simulink model "TLfaultDetection"  (R2024b)
settings: Solver=VariableStepAuto  StartTime=0.0  StopTime=0.15  RelTol=1e-3
undefined symbols (not defined in the file or in its folder): D1, Delta
libraries: spsCurrentMeasurementLib x4, spsDistributedParametersLineLib x2, spsThreePhaseVIMeasurementLib x2, spsThreePhaseParallelRLCLoadLib x1, spsThreePhaseTransformerTwoWindingsLib x1, spsThreePhaseFaultLib x1, spsThreePhaseSourceLib x1, sps_lib x1
settings Model: Creator=tanyagupta  LastModifiedBy=tanyagupta

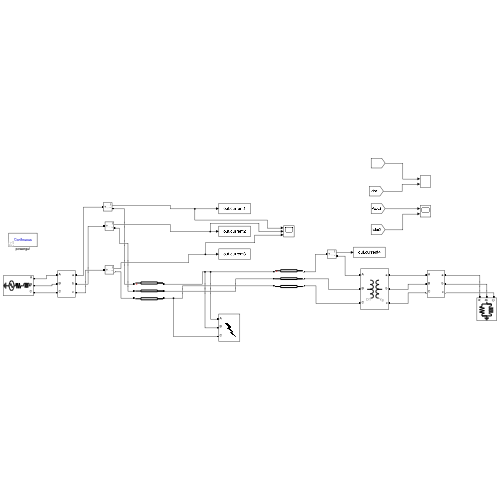
[thumbnail: Simulink's stored preview of the top-level diagram]
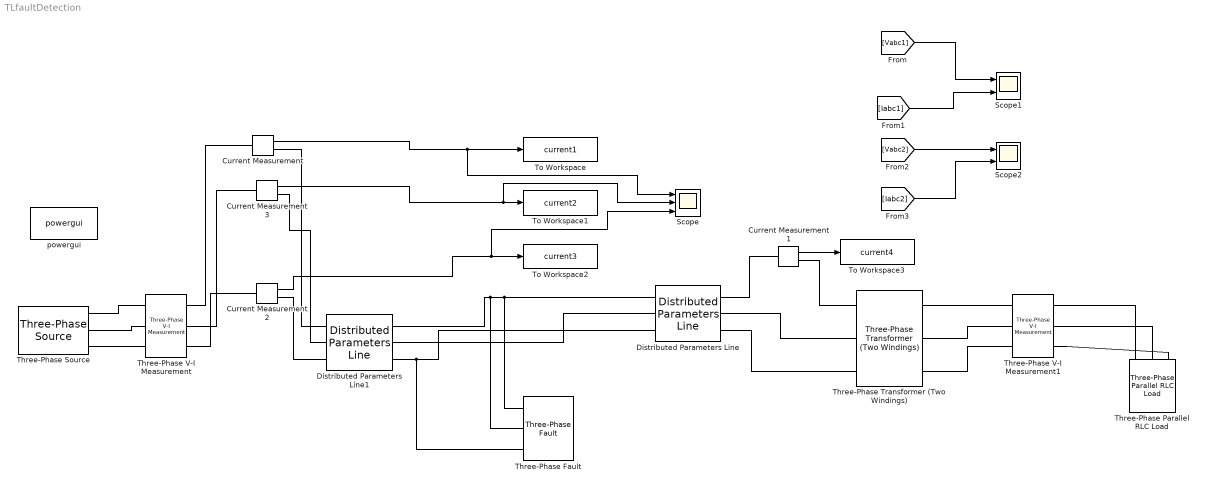
== system TLfaultDetection ==
  Current Measurement{,1..3} (4 alike) : spsCurrentMeasurementLib/Current Measurement  PhasorSimulation=off  OutputType=Complex  PSBequivalent=0
  Distributed Parameters Line : spsDistributedParametersLineLib/Distributed Parameters Line  Phases=3  Length=50  Frequency=50  Resistance=[0.01273 0.3864]  Inductance="[0.9337e-3  4.1264e-3]"  Capacitance=[12.74e-9 7.751e-9]  x1=[0.643345203283032 10685.4721352616 10685.709534853;314.159265358979 314.159265358979 314.159265358979;-1.45046970678582 0.439350851081216 -1.13144785804626]  x2=[0.645891773744692 10433.2952782558 10433.5270752232;314.159265358979 314.159265358979 314.159265358979;-1.45164893849604 0.415479570865668 -1.15531913826181]  x3=[0.000867813395751373 26.7060474479639 26.7066407773627;314.159265358979 314.159265358979 314.159265358979;-1.53989669369652 1.06083449813002 -0.509964210997466]  x4=[0.000867835898926565 59.119202827283 59.1205162811399;314.159265358979 314.159265358979 314.159265358979;-1.45164893856299 0.119678624370484 -1.451120084757]  x5=0.000282770783497871  V1=[0.6433 1.069e+04 1.069e+04;314.2 314.2 314.2;-1.45 0.4394 -1.131]  V2=[0.6459 1.043e+04 1.043e+04;314.2 314.2 314.2;-1.452 0.4155 -1.155]  I1=[0.0008678 26.71 26.71;314.2 314.2 314.2;-1.54 1.061 -0.51]  I2=[0.0008678 59.12 59.12;314.2 314.2 314.2;-1.452 0.1197 -1.451]  nHarmo=1  Measurements=None  Decoupling=off  VsMag0=0  VrMag0=0  VsAngle0=0  VrAngle0=0  IsMag0=0  IrMag0=0  IsAngle0=0  IrAngle0=0
      settings: LibrarySourceBlock=sps_lib/Power Grid Elements/Distributed Parameters Line
  Distributed Parameters Line1 : spsDistributedParametersLineLib/Distributed Parameters Line  Phases=3  Length=50  Frequency=50  Resistance=[0.01273 0.3864]  Inductance="[0.9337e-3  4.1264e-3]"  Capacitance=[12.74e-9 7.751e-9]  x1=[0.046718750025175 10912.2405740075 10912.3023533772;314.159265358979 314.159265358979 314.159265358979;-1.33974738551978 0.462312918608127 -1.10848469097388]  x2=[0.643345203283101 10685.4721352616 10685.709534853;314.159265358979 314.159265358979 314.159265358979;-1.45046970678603 0.439350851081216 -1.13144785804626]  x3=[0.0087348686824243 26.7149499857966 26.7084013172274;314.159265358979 314.159265358979 314.159265358979;-2.73368794344015 1.00510568053713 -0.566067723751181]  x4=[0.00848448242707922 59.1814937211343 59.1795703862869;314.159265358979 314.159265358979 314.159265358979;0.304089852166746 0.173381387862149 -1.39721638237216]  x5=0.000282770783497871  V1=[0.04672 1.091e+04 1.091e+04;314.2 314.2 314.2;-1.34 0.4623 -1.108]  V2=[0.6433 1.069e+04 1.069e+04;314.2 314.2 314.2;-1.45 0.4394 -1.131]  I1=[0.008735 26.71 26.71;314.2 314.2 314.2;-2.734 1.005 -0.5661]  I2=[0.008484 59.18 59.18;314.2 314.2 314.2;0.3041 0.1734 -1.397]  nHarmo=1  Measurements=None  Decoupling=off  VsMag0=0  VrMag0=0  VsAngle0=0  VrAngle0=0  IsMag0=0  IrMag0=0  IsAngle0=0  IrAngle0=0
      settings: LibrarySourceBlock=sps_lib/Power Grid Elements/Distributed Parameters Line
  Scope : Scope  NumInputPorts=3
  Scope1 : Scope  NumInputPorts=2
  Scope2 : Scope  NumInputPorts=2
  Three-Phase Parallel RLC Load : spsThreePhaseParallelRLCLoadLib/Three-Phase Parallel RLC Load  LConnTagsString=A|B|C  Configuration=Y (grounded)  NominalVoltage=0.4e3  Vabc=[1e3 1e3 1e3]  Vabcp=[1e3 1e3 1e3]  NominalFrequency=50  UnbalancedPower=off  ActivePower=10e3  InductivePower=100  CapacitivePower=0  Pabc=[10e3 9e3 11e3]  QLabc=[100 90 110]  QCabc=[100 90 110]  Pabcp=[10e3 9e3 11e3]  QLabcp=[100 90 110]  QCabcp=[100 90 110]  Measurements=None  LoadType=constant Z
  Three-Phase Transformer (Two Windings) : spsThreePhaseTransformerTwoWindingsLib/Three-Phase Transformer (Two Windings)  Winding1Connection=Delta (D1)  Winding2Connection=Yg  CoreType=Three single-phase transformers  SetSaturation=off  Hysteresis=off  DataFile='hysteresis'  SetInitialFlux=off  Measurements=None  UNITS=pu  NominalPower=[ 100e6 , 50 ]  Winding1=[ 11e3 , 0.002 , 0.08 ]  Winding2=[ 0.4e3 , 0.002 , 0.08 ]  Rm=500  Lm=500  L0=0.5  Saturation=[ 0,0 ; 0.0024,1.2 ; 1.0,1.52 ]  InitialFluxes=[ 0.8 , -0.8 , 0.7 ]  BreakLoop=off  DiscreteSolver=Trapezoidal iterative  DataType=off  TransfoNumber=1
  Three-Phase V-I Measurement : spsThreePhaseVIMeasurementLib/Three-Phase V-I Measurement  VoltageMeasurement=phase-to-ground  SetLabelV=on  LabelV=Vabc1  Vpu=off  VpuLL=off  CurrentMeasurement=yes  SetLabelI=on  LabelI=Iabc1  Ipu=off  Pbase=100e6  Vbase=500e3  OutputType=Complex  PhasorSimulation=off  PSBequivalent=0
  Three-Phase V-I Measurement1 : spsThreePhaseVIMeasurementLib/Three-Phase V-I Measurement  VoltageMeasurement=phase-to-ground  SetLabelV=on  LabelV=Vabc2  Vpu=off  VpuLL=off  CurrentMeasurement=yes  SetLabelI=on  LabelI=Iabc2  Ipu=off  Pbase=100e6  Vbase=500e3  OutputType=Complex  PhasorSimulation=off  PSBequivalent=0
  Three-Phase Fault : spsThreePhaseFaultLib/Three-Phase Fault  InitialStates=0  FaultA=off  FaultB=on  FaultC=off  GroundFault=on  SwitchTimes="[1/60  5/60]"  External=off  SwitchStatus=NaN  FaultResistance=0.001  GroundResistance=0.01  SnubberResistance=1e6  SnubberCapacitance=inf  Measurements=None
  Three-Phase Source : spsThreePhaseSourceLib/Three-Phase Source  InternalConnection=Yg  VoltagePhases=off  Voltage=11e3  PhaseAngle=0  Voltage_phases=[25e3 25e3 25e3]/sqrt(3)  PhaseAngles_phases=[0 -120 +120]  Frequency=50  NonIdealSource=on  SpecifyImpedance=off  Resistance=0.8929  Inductance=16.58e-3  ShortCircuitLevel=100e6  BaseVoltage=11e3  XRratio=7  BusType=swing  Pref=10e3  Qref=0  Prefabc=[10e3, 10e3, 10e3]  Qrefabc=[0, 0, 0]  Qmin=-inf  Qmax=inf
  To Workspace : ToWorkspace  VariableName=current1  SaveFormat=Structure With Time  SampleTime=-1
  To Workspace1 : ToWorkspace  VariableName=current2  SaveFormat=Structure With Time  SampleTime=-1
  To Workspace2 : ToWorkspace  VariableName=current3  SaveFormat=Structure With Time  SampleTime=-1
  To Workspace3 : ToWorkspace  VariableName=current4  SaveFormat=Structure With Time  SampleTime=-1
  powergui : sps_lib/powergui  Priority=1  SimulationMode=Continuous  SampleTime=50e-6  frequency=60  Iterations=50  frequencyindice=50  Pbase=100e6  ErrMax=1e-4  UnitsV=kV  UnitsW=MW  buscounter=0  FunctionMessages=off  echomessages=off  EnableUseOfTLC=off  CurrentSourceSwitches=on  DisableSnubberDevices=off  DisableRonSwitches=off  DisableVfSwitches=off  DisplayEquations=off  AutomaticDiscreteSolvers=off  SolverType=Tustin/Backward Euler (TBE)  Interpol=off  ExternalGateDelay=off  methode=off  Ts=100  x0status=blocks  SPID=on  SwTol=0  HookPort=off  NonlinearTolerance=1e-4  nMaxIteration=100  ContinueOnMaxIteration=off  RestoreLinks=warning  ResistiveCurrentMeasurement=off  Frange=[0:2:500]  Ylog=off  Xlog=on  ShowGrid=off  save=off  variable=ZData  structure=0  ZoomFFT=off  StartTime=0.0  cycles=1  DisplayStyle=1  fundamental=60  FreqAxis=off  MaxFrequency=1000  frequencyindicesteady=1  RmsSteady=1  display=off
  wires:
  Current Measurement3/1 -> Scope/2, To Workspace1/1
  Current Measurement2/1 -> Scope/3, To Workspace2/1
  Current Measurement/1 -> Scope/1, To Workspace/1
  Current Measurement1/1 -> To Workspace3/1
  [Vabc1] -> Scope1/1
  [Iabc1] -> Scope1/2
  [Vabc2] -> Scope2/1
  [Iabc2] -> Scope2/2
  connections:
  Three-Phase Source/RConn1 -- Three-Phase V-I Measurement/LConn1
  Three-Phase Source/RConn2 -- Three-Phase V-I Measurement/LConn2
  Three-Phase Source/RConn3 -- Three-Phase V-I Measurement/LConn3
  Three-Phase V-I Measurement/RConn1 -- Current Measurement/LConn1
  Three-Phase V-I Measurement/RConn2 -- Current Measurement3/LConn1
  Three-Phase V-I Measurement/RConn3 -- Current Measurement2/LConn1
  Current Measurement/RConn1 -- Distributed Parameters Line1/LConn1
  Current Measurement3/RConn1 -- Distributed Parameters Line1/LConn2
  Current Measurement2/RConn1 -- Distributed Parameters Line1/LConn3
  Current Measurement1/RConn1 -- Three-Phase Transformer (Two Windings)/LConn1
  Distributed Parameters Line1/RConn1 -- Three-Phase Fault/LConn2 -- Distributed Parameters Line/LConn1 -- Three-Phase Fault/LConn1
  Distributed Parameters Line1/RConn2 -- Distributed Parameters Line/LConn2
  Distributed Parameters Line1/RConn3 -- Three-Phase Fault/LConn3 -- Distributed Parameters Line/LConn3
  Distributed Parameters Line/RConn1 -- Current Measurement1/LConn1
  Distributed Parameters Line/RConn2 -- Three-Phase Transformer (Two Windings)/LConn2
  Distributed Parameters Line/RConn3 -- Three-Phase Transformer (Two Windings)/LConn3
  Three-Phase Transformer (Two Windings)/RConn2 -- Three-Phase V-I Measurement1/LConn2
  Three-Phase Transformer (Two Windings)/RConn1 -- Three-Phase V-I Measurement1/LConn1
  Three-Phase Transformer (Two Windings)/RConn3 -- Three-Phase V-I Measurement1/LConn3
  Three-Phase V-I Measurement1/RConn1 -- Three-Phase Parallel RLC Load/LConn1
  Three-Phase V-I Measurement1/RConn2 -- Three-Phase Parallel RLC Load/LConn2
  Three-Phase V-I Measurement1/RConn3 -- Three-Phase Parallel RLC Load/LConn3
